simulink model "p1"  (R2020a)
settings: Solver=VariableStepAuto  StartTime=0.0  StopTime=10.0  RelTol=1e-3
settings Model: Creator=007  LastModifiedBy=007

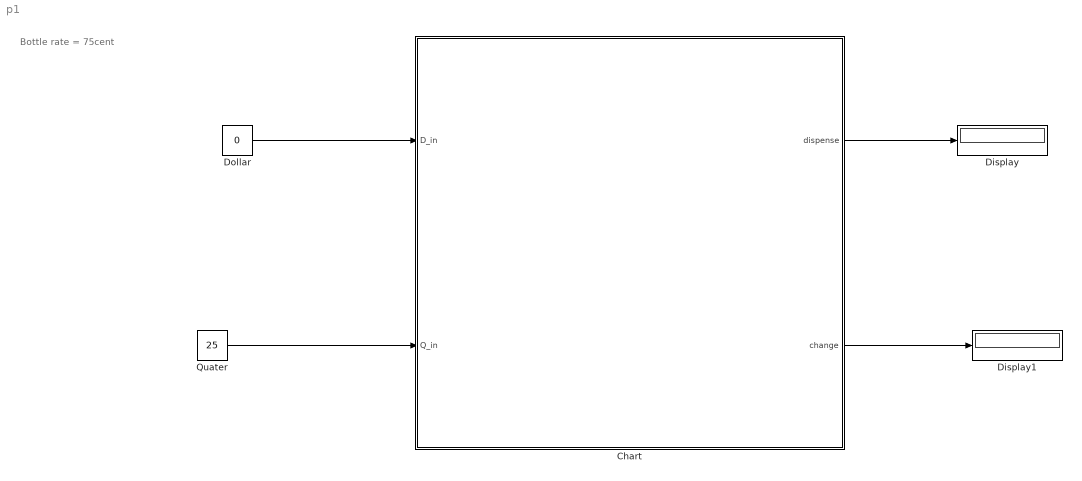
== system p1 ==
  note: Bottle rate = 75cent
  Chart : Stateflow chart  TreatAsAtomicUnit=on
  Display : Display
  Display1 : Display
  Dollar : Constant  Value=0
  Quater : Constant  Value=25
  wires:
  Chart/1(dispense) -> Display/1
  Quater/1 -> Chart/2(Q_in)
  Chart/2(change) -> Display1/1
  Dollar/1 -> Chart/1(D_in)

== stateflow chart p1/Chart ==
  note: WATER DISPENSING MACHINE
  state wait
  state cent25
  state cent50
  (default) -> wait
  wait -> wait [order 1] : [D_in==1]{dispense=1,change=25;}
  cent50 -> wait : [Q_in==25]{dispense=1,change=0;}
  wait -> cent25 [order 2] : [Q_in==25]{dispense=0,change=0;}
  cent25 -> cent50 : [Q_in==25]{dispense=0,change=0;}
  data: dispense output; change output; D_in input; Q_in input
